simulink model "Navion_6DoF_YANG"  (Simulink 10.3)
settings: Solver=ode45  StartTime=0.0  StopTime=100.0  FixedStep=.01  MaxStep=.004  RelTol=1e-5  EnableMultiTasking=on
values from neighbouring files (symbols this model uses):
  ac = [0 0 0]    [Navion_Geom6dof.m]
  b = 44    [Navion_Geom6dof.m]
  cbar = 4+2/12    (= 4.16666666667)    [Navion_Geom6dof.m]
  cda2 = 0.33    [Navion_Geom6dof.m]
  cdo = 0.05    [Navion_Geom6dof.m]
  cg = [0 0 0]    [Navion_Geom6dof.m]
  cla = 4.44    [Navion_Geom6dof.m]
  cladot = 0    [Navion_Geom6dof.m]
  clb = -0.074    [Navion_Geom6dof.m]
  clda = -0.134    [Navion_Geom6dof.m]
  clde = 0.355    [Navion_Geom6dof.m]
  cldr = 0.107    [Navion_Geom6dof.m]
  clo = 0.41    [Navion_Geom6dof.m]
  clp = -0.410    (= -0.41)    [Navion_Geom6dof.m]
  clq = 3.8    [Navion_Geom6dof.m]
  clr = 0.107    [Navion_Geom6dof.m]
  cma = -0.683    [Navion_Geom6dof.m]
  cmadot = -4.36    [Navion_Geom6dof.m]
  cmde = -0.923    [Navion_Geom6dof.m]
  cmq = -9.96    [Navion_Geom6dof.m]
  cnb = 0.071    [Navion_Geom6dof.m]
  cnda = -0.0035    [Navion_Geom6dof.m]
  cndr = -0.072    [Navion_Geom6dof.m]
  cnp = -0.0575    [Navion_Geom6dof.m]
  cnr = -0.125    [Navion_Geom6dof.m]
  cyb = -0.564    [Navion_Geom6dof.m]
  cydr = 0.157    [Navion_Geom6dof.m]
  initalt = 6000    [Navion_Geom6dof.m]
  initbank = 0    [Navion_Geom6dof.m]
  initeast = 0    [Navion_Geom6dof.m]
  inithead = 0    [Navion_Geom6dof.m]
  initnorth = 0    [Navion_Geom6dof.m]
  initp = 0    [Navion_Geom6dof.m]
  initpitch = initw/initu    (= -0.0290599038041)    [Navion_Geom6dof.m]
  initq = 0    [Navion_Geom6dof.m]
  initr = 0    [Navion_Geom6dof.m]
  initu = 228.7    [Navion_Geom6dof.m]
  initv = 0    [Navion_Geom6dof.m]
  initw = -6.646    [Navion_Geom6dof.m]
  jx = 1048    [Navion_Geom6dof.m]
  jxz = 0    [Navion_Geom6dof.m]
  jy = 3000    [Navion_Geom6dof.m]
  jz = 3500    [Navion_Geom6dof.m]
  Pos_L = [95.46/12-3.882,5.1875,0]    [Navion_Geom6dof.m]
  Pos_R = [95.46/12,-5.1875,0]    [Navion_Geom6dof.m]
  sw = 175.3    [Navion_Geom6dof.m]
  Vect_L = [0.998,-0.057,0.017]    [Navion_Geom6dof.m]
  Vect_R = [0.998,0.057,0.017]    [Navion_Geom6dof.m]
  weight = 3695    [Navion_Geom6dof.m]
undefined symbols (not defined in the file or in its folder): BHP_A, BHP_B, CP_norm, Pr_Alt, PropEff_norm
libraries: simulink_extras x4, aerolibatmos2 x2
(part 1 of 2)
settings Model: Creator=andersop  LastModifiedBy=YANGX5  MultithreadedSim=on  ExtModeAutoUpdateStatusClock=off
settings SolverCC: InitialStep=.004
settings DataIOCC: LimitDataPoints=on  SaveState=on  SignalLoggingName=sigsOut
settings OptimizationCC: InitFltsAndDblsToZero=on
settings DebuggingCC: SaveWithParameterizedLinksMsg=none  SignalResolutionControl=TryResolveAllWithWarning  MultiTaskDSMMsg=warning  MultiTaskCondExecSysMsg=none
settings HardwareCC: TargetUnknown=on
settings GRTTargetCC: TargetFcnLib=ansi_tfl_tmw.mat  ModelReferenceCompliant=off  MatFileLogging=off

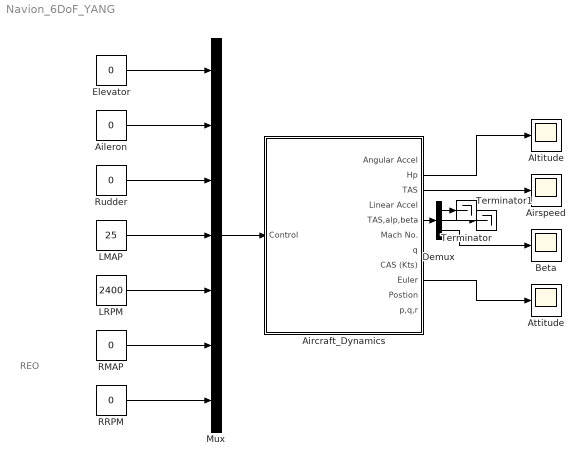
== system Navion_6DoF_YANG ==
  note: REO
  Aileron : Constant  Value=0
  Aircraft_Dynamics : Subsystem
  Airspeed : Scope
  Altitude : Scope
  Attitude : Scope
  Beta : Scope
  Demux : Demux  Outputs=3
  Elevator : Constant  Value=0
  LMAP : Constant  Value=25
  LRPM : Constant  Value=2400
  Mux : Mux  Inputs=7
  RMAP : Constant  Value=0
  RRPM : Constant  Value=0
  Rudder : Constant  Value=0
  Terminator : Terminator
  Terminator1 : Terminator
  wires:
  Mux/1 -> Aircraft_Dynamics/1(Control)
  Elevator/1 -> Mux/1
  LRPM/1 -> Mux/5
  RMAP/1 -> Mux/6
  RRPM/1 -> Mux/7
  Aileron/1 -> Mux/2
  Rudder/1 -> Mux/3
  LMAP/1 -> Mux/4
  Aircraft_Dynamics/2(Hp) -> Altitude/1
  Aircraft_Dynamics/3(TAS) -> Airspeed/1
  Aircraft_Dynamics/9(Euler) -> Attitude/1
  Aircraft_Dynamics/5(TAS,alp,beta) -> Demux/1
  Demux/3 -> Beta/1
  Demux/1 -> Terminator/1
  Demux/2 -> Terminator1/1

== system Navion_6DoF_YANG/Aircraft_Dynamics ==
  Control : Inport
  Aerodynamics : Subsystem
  Display : Display
  Engines : Subsystem
  "Equations of motion numerical integration " : Subsystem
  Flight Parameters : Subsystem
  Linear Acc and Moments : Subsystem
  "Mass, CG & inertia" : Subsystem
  Standard Atmosphere : Subsystem
  Angular Accel : Outport
  Hp : Outport  Port=2
  TAS : Outport  Port=3
  Linear Accel : Outport  Port=4
  TAS,alp,beta : Outport  Port=5
  Mach No. : Outport  Port=6
  q : Outport  Port=7
  CAS (Kts) : Outport  Port=8
  Euler : Outport  Port=9
  Postion : Outport  Port=10
  p,q,r : Outport  Port=11
  wires:
  Aerodynamics/1(Faero) -> Linear Acc and Moments/1(Faero)
  Aerodynamics/2(Maero) -> Linear Acc and Moments/2(Maero)
  Control/1 -> Aerodynamics/3(Controls), Engines/1(Control)
  "Mass, CG & inertia"/1(CG) -> Linear Acc and Moments/6(CG)
  "Mass, CG & inertia"/2(Inertia) -> "Equations of motion numerical integration "/2(Inertia)
  Linear Acc and Moments/1(Lin Accel) -> Linear Accel/1, "Equations of motion numerical integration "/1(Accel)
  Linear Acc and Moments/2(Moments) -> "Equations of motion numerical integration "/3(Moments)
  "Equations of motion numerical integration "/3(Ang rates) -> Aerodynamics/6(p,q,r), p,q,r/1
  "Equations of motion numerical integration "/4(Wind Vel) -> Flight Parameters/1(Wind Vel), Display/1
  Flight Parameters/1(Wing Para) -> TAS,alp,beta/1, Aerodynamics/1(Wind Para), Engines/2(Wind Par)
  Flight Parameters/4(Dyn (q)) -> Aerodynamics/2(dyn(q)), q/1
  Flight Parameters/3(Mach No.) -> Mach No./1, Aerodynamics/4(Mach No.)
  Flight Parameters/2(A&Bdot) -> Aerodynamics/5(a&bdot)
  "Equations of motion numerical integration "/2(Position) -> Postion/1, Standard Atmosphere/1(Position)
  "Equations of motion numerical integration "/1(Ang Accel) -> Angular Accel/1
  Standard Atmosphere/4(Hp) -> Engines/3(Hp), Hp/1
  Flight Parameters/5(TAS fps) -> TAS/1
  Flight Parameters/6(CAS(kts)) -> CAS (Kts)/1
  "Equations of motion numerical integration "/5(Euler) -> Euler/1
  Standard Atmosphere/3(a) -> Flight Parameters/2(a)
  Standard Atmosphere/2(rho) -> Flight Parameters/3(rho)
  "Mass, CG & inertia"/3(mass) -> Linear Acc and Moments/5(Mass)
  Standard Atmosphere/1(OAT) -> Engines/4(OTA)
  Engines/1(Feng_L) -> Linear Acc and Moments/3(Feng_L)
  Engines/2(Feng_R) -> Linear Acc and Moments/4(Feng_R)

== system Navion_6DoF_YANG/Aircraft_Dynamics/Aerodynamics ==
  note: Notes: alpha is measured from
  Wind Para : Inport
  dyn(q) : Inport  Port=2
  Controls : Inport  Port=3
  Mach No. : Inport  Port=4
  a&bdot : Inport  Port=5
  p,q,r : Inport  Port=6
  Aero Forces and Moments : Subsystem
  CD : Subsystem
  CL : Subsystem
  CM : Subsystem
  CN : Subsystem
  CY : Subsystem
  Croll : Subsystem
  Faero : Outport
  Maero : Outport  Port=2
  wires:
  Wind Para/1 -> CL/1(Wind Parameters), CY/1(Wind Parameters), Aero Forces and Moments/5(Wind Para), CN/1(Wind Parameters), Croll/1(Wind Parameters), CM/1(Wind Parameters), CD/1(Wind Parameters)
  CL/1(CL) -> Aero Forces and Moments/4(CL)
  Mach No./1 -> CM/3(Mach No.), CN/3(Mach No.), Croll/3(Mach No.), CY/3(Mach No.), CL/3(Mach No.), CD/3(Mach No.)
  a&bdot/1 -> CL/4(a&bdot), CM/4(a&bdot)
  p,q,r/1 -> CM/5(P,q,r), CN/4(P,q,r), Croll/4(P,q,r), CY/4(P,q,r), CL/5(P,q,r)
  Controls/1 -> CM/2(Controls), CD/2(Controls), CN/2(Controls), Croll/2(Controls), CY/2(Controls), CL/2(Controls)
  CD/1(CD) -> Aero Forces and Moments/2(CD)
  CN/1(CN) -> Aero Forces and Moments/8(CN)
  Croll/1(Croll) -> Aero Forces and Moments/6(Croll)
  CY/1(CY) -> Aero Forces and Moments/3(CY)
  CM/1(CM) -> Aero Forces and Moments/7(CM)
  dyn(q)/1 -> Aero Forces and Moments/1(dyn(q))
  Aero Forces and Moments/1(Faero) -> Faero/1
  Aero Forces and Moments/2(Maero) -> Maero/1

== system Navion_6DoF_YANG/Aircraft_Dynamics/Engines ==
  Control : Inport
  Wind Par : Inport  Port=2
  Hp : Inport  Port=3
  OTA : Inport  Port=4
  Demux : Demux  Outputs=7
  Demux1 : Demux  Outputs=3
  Display : Display
  Display1 : Display
  Lycoming IO-Left : Subsystem
  Lycoming IO-Right : Subsystem
  Terminator{,1..4} (5 alike) : Terminator
  Feng_L : Outport
  Feng_R : Outport  Port=2
  tag scope: TAS=global
  wires:
  Control/1 -> Demux/1
  Demux/1 -> Terminator/1
  Demux/2 -> Terminator1/1
  Demux/3 -> Terminator2/1
  Lycoming IO-Left/1(Thrust Left) -> Feng_L/1, Display/1
  Wind Par/1 -> Demux1/1
  Demux1/2 -> Terminator4/1
  Demux1/3 -> Terminator3/1
  Lycoming IO-Right/1(Thrust right) -> Feng_R/1, Display1/1
  Demux/4 -> Lycoming IO-Left/1(MAP_L)
  Demux/5 -> Lycoming IO-Left/2(RPM_L)
  Demux/6 -> Lycoming IO-Right/1(MAP_R)
  Demux/7 -> Lycoming IO-Right/2(RPM_R)
  Hp/1 -> Lycoming IO-Right/3(Press alt), Lycoming IO-Left/3(Press alt)
  OTA/1 -> Lycoming IO-Right/4(Inlt Temp), Lycoming IO-Left/4(Inlt Temp)
  Demux1/1 -> [TAS]  "TAS"

== system Navion_6DoF_YANG/Aircraft_Dynamics/Equations of motion numerical integration  ==
  Accel : Inport
  Inertia : Inport  Port=2
  Moments : Inport  Port=3
  Flat Earth Navigation : Subsystem
  Force Equations : Subsystem
  Gravity Model : Subsystem
  Inert-body : Subsystem
  Kinematic Equiations : Subsystem
  Moment Equations : Subsystem
  Ang Accel : Outport
  Position : Outport  Port=2
  Ang rates : Outport  Port=3
  Wind Vel : Outport  Port=4
  Euler : Outport  Port=5
  wires:
  Moment Equations/1(Ang Rates) -> Kinematic Equiations/1(Rates), Force Equations/3(Rates), Ang rates/1
  Kinematic Equiations/1(Euler angles) -> Flat Earth Navigation/1(Euler Angles), Inert-body/1(Euler), Euler/1
  Force Equations/1(Lin Vel) -> Wind Vel/1, Flat Earth Navigation/2(Velocity)
  Accel/1 -> Force Equations/1(Accel)
  Inertia/1 -> Moment Equations/1(Inertia)
  Gravity Model/1(Gravity) -> Force Equations/2(Gravity)
  Moments/1 -> Moment Equations/2(Moments)
  Moment Equations/2(Ang Accel) -> Ang Accel/1
  Flat Earth Navigation/1(Position) -> Position/1
  Inert-body/1(NEDtoBC) -> Force Equations/4(NEDtoABC)

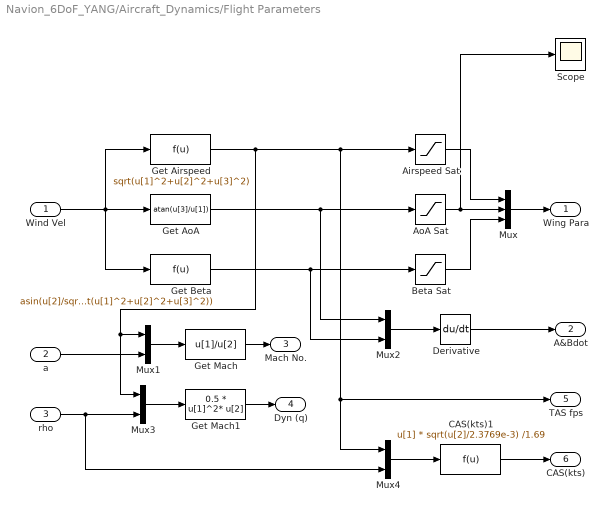
== system Navion_6DoF_YANG/Aircraft_Dynamics/Flight Parameters ==
  Wind Vel : Inport
  a : Inport  Port=2
  rho : Inport  Port=3
  Airspeed Sat : Saturate  UpperLimit=1100  LowerLimit=0
  AoA Sat : Saturate  UpperLimit=0.3  LowerLimit=-0.2
  Beta Sat : Saturate  UpperLimit=0.4  LowerLimit=-0.4
  CAS(kts)1 : Fcn  Expr=u[1] * sqrt(u[2]/2.3769e-3) /1.69
  Derivative : Derivative
  Get Airspeed : Fcn  Expr=sqrt(u[1]^2+u[2]^2+u[3]^2)
  Get AoA : Fcn  Expr=atan(u[3]/u[1])
  Get Beta : Fcn  Expr=asin(u[2]/sqrt(u[1]^2+u[2]^2+u[3]^2))
  Get Mach : Fcn  Expr=u[1]/u[2]
  Get Mach1 : Fcn  Expr=0.5 * u[1]^2* u[2]
  Mux : Mux  Inputs=3
  Mux{1..4} (4 alike) : Mux  Inputs=2
  Scope : Scope
  Wing Para : Outport
  A&Bdot : Outport  Port=2
  Mach No. : Outport  Port=3
  Dyn (q) : Outport  Port=4
  TAS fps : Outport  Port=5
  CAS(kts) : Outport  Port=6
  wires:
  Wind Vel/1 -> Get AoA/1, Get Airspeed/1, Get Beta/1
  Get Airspeed/1 -> Mux1/1, Mux3/1, Airspeed Sat/1, TAS fps/1, Mux4/1
  Get AoA/1 -> AoA Sat/1, Mux2/1
  Get Beta/1 -> Beta Sat/1, Mux2/2
  AoA Sat/1 -> Mux/2, Scope/1
  Airspeed Sat/1 -> Mux/1
  Beta Sat/1 -> Mux/3
  Mux/1 -> Wing Para/1
  Mux1/1 -> Get Mach/1
  a/1 -> Mux1/2
  Mux2/1 -> Derivative/1
  Derivative/1 -> A&Bdot/1
  Get Mach/1 -> Mach No./1
  rho/1 -> Mux3/2, Mux4/2
  Mux3/1 -> Get Mach1/1
  Get Mach1/1 -> Dyn (q)/1
  Mux4/1 -> CAS(kts)1/1
  CAS(kts)1/1 -> CAS(kts)/1

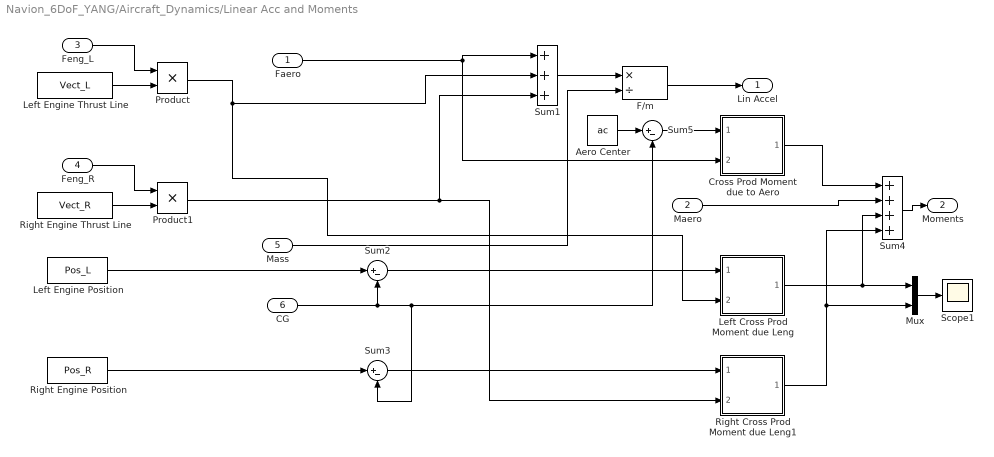
== system Navion_6DoF_YANG/Aircraft_Dynamics/Linear Acc and Moments ==
  Faero : Inport
  Maero : Inport  Port=2
  Feng_L : Inport  Port=3
  Feng_R : Inport  Port=4
  Mass : Inport  Port=5
  CG : Inport  Port=6
  Aero Center : Constant  Value=ac
  Cross Prod Moment due to Aero : Subsystem
  F/m : Product  Inputs=*/  SaturateOnIntegerOverflow=on  OutDataTypeStr=Inherit: Same as first input
  Left Cross Prod Moment due Leng : Subsystem
  Left Engine Position : Constant  Value=Pos_L
  Left Engine Thrust Line : Constant  Value=Vect_L
  Mux : Mux  Inputs=2
  Product : Product
  Product1 : Product
  Right Cross Prod Moment due Leng1 : Subsystem
  Right Engine Position : Constant  Value=Pos_R
  Right Engine Thrust Line : Constant  Value=Vect_R
  Scope1 : Scope
  Sum1 : Sum  Inputs=+++  SaturateOnIntegerOverflow=on
  Sum2 : Sum  Inputs=|+-  SaturateOnIntegerOverflow=on
  Sum3 : Sum  Inputs=|+-  SaturateOnIntegerOverflow=on
  Sum4 : Sum  Inputs=++++  SaturateOnIntegerOverflow=on
  Sum5 : Sum  Inputs=|+-  SaturateOnIntegerOverflow=on
  Lin Accel : Outport
  Moments : Outport  Port=2
  wires:
  Product/1 -> Sum1/2, Left Cross Prod Moment due Leng/2(Vec 2)
  Faero/1 -> Sum1/1, Cross Prod Moment due to Aero/2(Vec 2)
  Sum1/1 -> F/m/1
  Mass/1 -> F/m/2
  F/m/1 -> Lin Accel/1
  Aero Center/1 -> Sum5/1
  Sum5/1 -> Cross Prod Moment due to Aero/1(Vec 1)
  Maero/1 -> Sum4/2
  Sum4/1 -> Moments/1
  Cross Prod Moment due to Aero/1(X Prod) -> Sum4/1
  Sum2/1 -> Left Cross Prod Moment due Leng/1(Vec 1)
  Left Cross Prod Moment due Leng/1(X Prod) -> Mux/1, Sum4/3
  Left Engine Position/1 -> Sum2/1
  Feng_L/1 -> Product/1
  Left Engine Thrust Line/1 -> Product/2
  Feng_R/1 -> Product1/1
  Right Engine Thrust Line/1 -> Product1/2
  Right Engine Position/1 -> Sum3/1
  CG/1 -> Sum2/2, Sum3/2, Sum5/2
  Sum3/1 -> Right Cross Prod Moment due Leng1/1(Vec 1)
  Product1/1 -> Sum1/3, Right Cross Prod Moment due Leng1/2(Vec 2)
  Right Cross Prod Moment due Leng1/1(X Prod) -> Mux/2, Sum4/4
  Mux/1 -> Scope1/1

== system Navion_6DoF_YANG/Aircraft_Dynamics/Mass, CG & inertia ==
  Mux1 : Mux
  cg : Constant  Value=cg
  jx : Constant  Value=jx
  jxz : Constant  Value=jxz
  jy : Constant  Value=jy
  jz : Constant  Value=jz
  mass2 : Constant  Value=weight/32.2
  CG : Outport
  Inertia : Outport  Port=2
  mass : Outport  Port=3
  wires:
  cg/1 -> CG/1
  jy/1 -> Mux1/2
  jx/1 -> Mux1/1
  jz/1 -> Mux1/3
  jxz/1 -> Mux1/4
  Mux1/1 -> Inertia/1
  mass2/1 -> mass/1

== system Navion_6DoF_YANG/Aircraft_Dynamics/Standard Atmosphere ==
  Position : Inport
  Demux : Demux  Outputs=3
      settings: DisplayOption=none
  Density : Fcn  Expr=2.3769e-3*(1 - 0.703e-5 * u[1])^4.14
  OATemp : Lookup  InputValues=[0 35000 60000]  Table=[519 390 390]  SaturateOnIntegerOverflow=on
  Speed of Sound : Fcn  Expr=sqrt(1.4*1716.3*u[1])
  Terminator : Terminator
  Terminator1 : Terminator
  OAT : Outport
  rho : Outport  Port=2
  a : Outport  Port=3
  Hp : Outport  Port=4
  wires:
  OATemp/1 -> OAT/1, Speed of Sound/1
  Density/1 -> rho/1
  Speed of Sound/1 -> a/1
  Position/1 -> Demux/1
  Demux/1 -> Terminator/1
  Demux/2 -> Terminator1/1
  Demux/3 -> OATemp/1, Density/1, Hp/1

== system Navion_6DoF_YANG/Aircraft_Dynamics/Aerodynamics/Aero Forces and Moments ==
  dyn(q) : Inport
  CD : Inport  Port=2
  CY : Inport  Port=3
  CL : Inport  Port=4
  Wind Para : Inport  Port=5
  Croll : Inport  Port=6
  CM : Inport  Port=7
  CN : Inport  Port=8
  Aerodynamic Forces : Subsystem
  Aerodynamic Moments : Subsystem
  Faero : Outport
  Maero : Outport  Port=2
  wires:
  dyn(q)/1 -> Aerodynamic Moments/1(dyn(q)), Aerodynamic Forces/5(dyn(q))
  CD/1 -> Aerodynamic Forces/1(CD)
  CY/1 -> Aerodynamic Forces/2(CY)
  CL/1 -> Aerodynamic Forces/3(CL)
  Wind Para/1 -> Aerodynamic Forces/4(Wind Para)
  Croll/1 -> Aerodynamic Moments/2(Croll)
  CM/1 -> Aerodynamic Moments/3(CM)
  CN/1 -> Aerodynamic Moments/4(CN)
  Aerodynamic Forces/1(FaeroBody) -> Faero/1
  Aerodynamic Moments/1(Maero) -> Maero/1

== system Navion_6DoF_YANG/Aircraft_Dynamics/Aerodynamics/CD ==
  Wind Parameters : Inport
  Controls : Inport  Port=2
  Mach No. : Inport  Port=3
  "   1" : Terminator
  "   6" : Terminator
  Get Alpha : Subsystem
  Math Function : Math  Operator=square  SignedPower=on  SaturateOnIntegerOverflow=on
  Sum : Sum  SaturateOnIntegerOverflow=on
  cda2 : Gain  Gain=cda2  SaturateOnIntegerOverflow=on  OutDataTypeStr=Inherit: Same as input  ParamDataTypeStr=Inherit: Same as input
  cdo : Constant  Value=cdo
  CD : Outport
  wires:
  Wind Parameters/1 -> Get Alpha/1(windPar)
  Sum/1 -> CD/1
  Controls/1 -> "   6"/1
  Get Alpha/1(Alpha) -> Math Function/1
  Math Function/1 -> cda2/1
  cda2/1 -> Sum/2
  Mach No./1 -> "   1"/1
  cdo/1 -> Sum/1

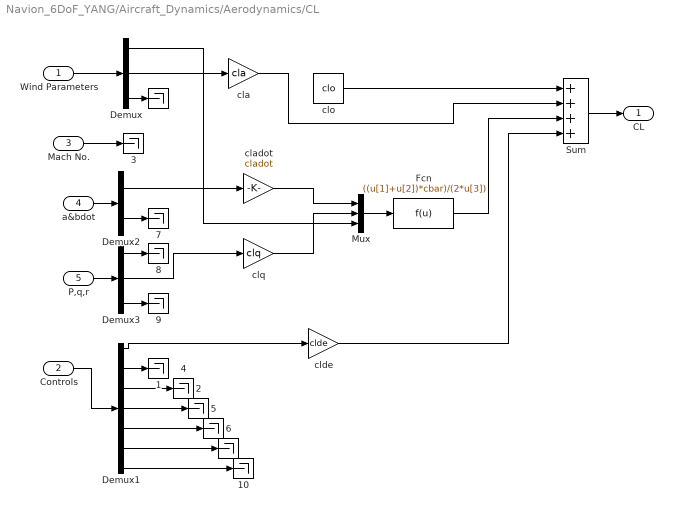
== system Navion_6DoF_YANG/Aircraft_Dynamics/Aerodynamics/CL ==
  Wind Parameters : Inport
  Controls : Inport  Port=2
  Mach No. : Inport  Port=3
  a&bdot : Inport  Port=4
  P,q,r : Inport  Port=5
     {,1..10} (11 alike) : Terminator
  Demux : Demux  Outputs=3
      settings: DisplayOption=none
  Demux1 : Demux  Outputs=7
      settings: DisplayOption=none
  Demux2 : Demux  Outputs=2
      settings: DisplayOption=none
  Demux3 : Demux  Outputs=3
      settings: DisplayOption=none
  Fcn : Fcn  Expr=((u[1]+u[2])*cbar)/(2*u[3])
  Mux : Mux  Inputs=3
  Sum : Sum  Inputs=++++  SaturateOnIntegerOverflow=on
  cla : Gain  Gain=cla  SaturateOnIntegerOverflow=on  OutDataTypeStr=Inherit: Same as input  ParamDataTypeStr=Inherit: Same as input
  cladot : Gain  Gain=cladot  SaturateOnIntegerOverflow=on  OutDataTypeStr=Inherit: Same as input  ParamDataTypeStr=Inherit: Same as input
  clde : Gain  Gain=clde  SaturateOnIntegerOverflow=on  OutDataTypeStr=Inherit: Same as input  ParamDataTypeStr=Inherit: Same as input
  clo : Constant  Value=clo
  clq : Gain  Gain=clq  SaturateOnIntegerOverflow=on  OutDataTypeStr=Inherit: Same as input  ParamDataTypeStr=Inherit: Same as input
  CL : Outport
  wires:
  Mux/1 -> Fcn/1
  Demux/1 -> Mux/3
  clo/1 -> Sum/1
  Demux2/2 -> "   7"/1
  Demux3/1 -> "   8"/1
  Demux3/3 -> "   9"/1
  Wind Parameters/1 -> Demux/1
  Sum/1 -> CL/1
  Controls/1 -> Demux1/1
  a&bdot/1 -> Demux2/1
  P,q,r/1 -> Demux3/1
  Demux/3 -> "   "/1
  Demux1/4 -> "   2"/1
  cla/1 -> Sum/2
  Demux2/1 -> cladot/1
  cladot/1 -> Mux/1
  Demux/2 -> cla/1
  clq/1 -> Mux/2
  Mach No./1 -> "   3"/1
  Demux3/2 -> clq/1
  Demux1/1 -> clde/1
  Demux1/2 -> "   1"/1
  Demux1/3 -> "   4"/1
  Fcn/1 -> Sum/3
  clde/1 -> Sum/4
  Demux1/5 -> "   5"/1
  Demux1/6 -> "   6"/1
  Demux1/7 -> "   10"/1

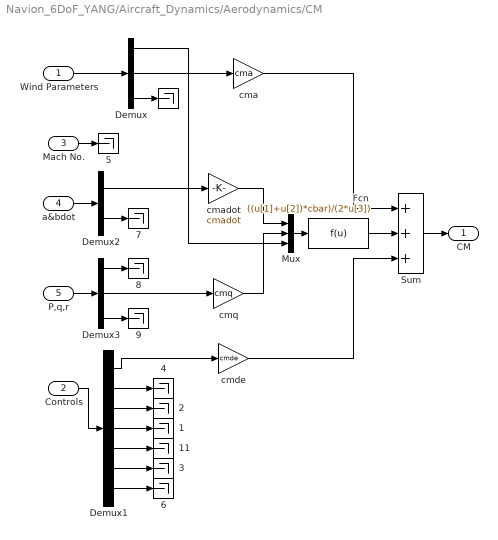
== system Navion_6DoF_YANG/Aircraft_Dynamics/Aerodynamics/CM ==
  Wind Parameters : Inport
  Controls : Inport  Port=2
  Mach No. : Inport  Port=3
  a&bdot : Inport  Port=4
  P,q,r : Inport  Port=5
     {,1..9,11} (11 alike) : Terminator
  Demux : Demux  Outputs=3
      settings: DisplayOption=none
  Demux1 : Demux  Outputs=7
      settings: DisplayOption=none
  Demux2 : Demux  Outputs=2
      settings: DisplayOption=none
  Demux3 : Demux  Outputs=3
      settings: DisplayOption=none
  Fcn : Fcn  Expr=((u[1]+u[2])*cbar)/(2*u[3])
  Mux : Mux  Inputs=3
  Sum : Sum  Inputs=+++  SaturateOnIntegerOverflow=on
  cma : Gain  Gain=cma  SaturateOnIntegerOverflow=on  OutDataTypeStr=Inherit: Same as input  ParamDataTypeStr=Inherit: Same as input
  cmadot : Gain  Gain=cmadot  SaturateOnIntegerOverflow=on  OutDataTypeStr=Inherit: Same as input  ParamDataTypeStr=Inherit: Same as input
  cmde : Gain  Gain=cmde  SaturateOnIntegerOverflow=on  OutDataTypeStr=Inherit: Same as input  ParamDataTypeStr=Inherit: Same as input
  cmq : Gain  Gain=cmq  SaturateOnIntegerOverflow=on  OutDataTypeStr=Inherit: Same as input  ParamDataTypeStr=Inherit: Same as input
  CM : Outport
  wires:
  Demux2/2 -> "   7"/1
  Demux3/1 -> "   8"/1
  Demux3/3 -> "   9"/1
  Wind Parameters/1 -> Demux/1
  Sum/1 -> CM/1
  Controls/1 -> Demux1/1
  a&bdot/1 -> Demux2/1
  P,q,r/1 -> Demux3/1
  Demux/3 -> "   "/1
  Demux1/4 -> "   1"/1
  Demux1/3 -> "   2"/1
  Demux/2 -> cma/1
  cmadot/1 -> Mux/1
  cmq/1 -> Mux/2
  Mux/1 -> Fcn/1
  Demux1/2 -> "   4"/1
  Mach No./1 -> "   5"/1
  Demux/1 -> Mux/3
  cma/1 -> Sum/1
  Demux1/1 -> cmde/1
  Demux2/1 -> cmadot/1
  Demux3/2 -> cmq/1
  Fcn/1 -> Sum/2
  cmde/1 -> Sum/3
  Demux1/5 -> "   11"/1
  Demux1/6 -> "   3"/1
  Demux1/7 -> "   6"/1

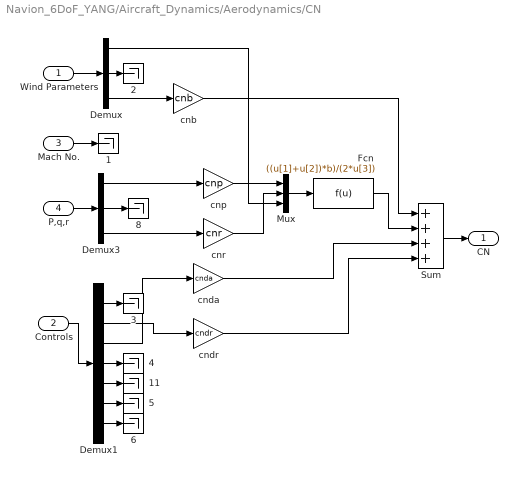
== system Navion_6DoF_YANG/Aircraft_Dynamics/Aerodynamics/CN ==
  Wind Parameters : Inport
  Controls : Inport  Port=2
  Mach No. : Inport  Port=3
  P,q,r : Inport  Port=4
     {1..6,8,11} (8 alike) : Terminator
  Demux : Demux  Outputs=3
      settings: DisplayOption=none
  Demux1 : Demux  Outputs=7
      settings: DisplayOption=none
  Demux3 : Demux  Outputs=3
      settings: DisplayOption=none
  Fcn : Fcn  Expr=((u[1]+u[2])*b)/(2*u[3])
  Mux : Mux  Inputs=3
  Sum : Sum  Inputs=++++  SaturateOnIntegerOverflow=on
  cnb : Gain  Gain=cnb  SaturateOnIntegerOverflow=on  OutDataTypeStr=Inherit: Same as input  ParamDataTypeStr=Inherit: Same as input
  cnda : Gain  Gain=cnda  SaturateOnIntegerOverflow=on  OutDataTypeStr=Inherit: Same as input  ParamDataTypeStr=Inherit: Same as input
  cndr : Gain  Gain=cndr  SaturateOnIntegerOverflow=on  OutDataTypeStr=Inherit: Same as input  ParamDataTypeStr=Inherit: Same as input
  cnp : Gain  Gain=cnp  SaturateOnIntegerOverflow=on  OutDataTypeStr=Inherit: Same as input  ParamDataTypeStr=Inherit: Same as input
  cnr : Gain  Gain=cnr  SaturateOnIntegerOverflow=on  OutDataTypeStr=Inherit: Same as input  ParamDataTypeStr=Inherit: Same as input
  CN : Outport
  wires:
  Mux/1 -> Fcn/1
  Demux/2 -> "   2"/1
  Wind Parameters/1 -> Demux/1
  Sum/1 -> CN/1
  Controls/1 -> Demux1/1
  P,q,r/1 -> Demux3/1
  Demux3/2 -> "   8"/1
  cnb/1 -> Sum/1
  Mach No./1 -> "   1"/1
  Demux/3 -> cnb/1
  Demux/1 -> Mux/3
  Demux3/1 -> cnp/1
  cnp/1 -> Mux/1
  Demux3/3 -> cnr/1
  cnr/1 -> Mux/2
  Demux1/2 -> cndr/1
  Demux1/3 -> cnda/1
  Fcn/1 -> Sum/2
  cnda/1 -> Sum/3
  cndr/1 -> Sum/4
  Demux1/1 -> "   3"/1
  Demux1/4 -> "   4"/1
  Demux1/5 -> "   11"/1
  Demux1/6 -> "   5"/1
  Demux1/7 -> "   6"/1

== system Navion_6DoF_YANG/Aircraft_Dynamics/Aerodynamics/CY ==
  Wind Parameters : Inport
  Controls : Inport  Port=2
  Mach No. : Inport  Port=3
  P,q,r : Inport  Port=4
     {1..5,8..12} (10 alike) : Terminator
  Demux : Demux  Outputs=3
      settings: DisplayOption=none
  Demux1 : Demux  Outputs=7
      settings: DisplayOption=none
  Sum : Sum  SaturateOnIntegerOverflow=on
  cyb : Gain  Gain=cyb  SaturateOnIntegerOverflow=on  OutDataTypeStr=Inherit: Same as input  ParamDataTypeStr=Inherit: Same as input
  cydr : Gain  Gain=cydr  SaturateOnIntegerOverflow=on  OutDataTypeStr=Inherit: Same as input  ParamDataTypeStr=Inherit: Same as input
  CY : Outport
  wires:
  Demux/2 -> "   9"/1
  Wind Parameters/1 -> Demux/1
  Sum/1 -> CY/1
  Controls/1 -> Demux1/1
  P,q,r/1 -> "   8"/1
  Demux/3 -> cyb/1
  Mach No./1 -> "   2"/1
  Demux1/1 -> "   10"/1
  Demux1/2 -> cydr/1
  Demux1/4 -> "   11"/1
  cyb/1 -> Sum/1
  cydr/1 -> Sum/2
  Demux/1 -> "   12"/1
  Demux1/3 -> "   1"/1
  Demux1/5 -> "   3"/1
  Demux1/6 -> "   4"/1
  Demux1/7 -> "   5"/1

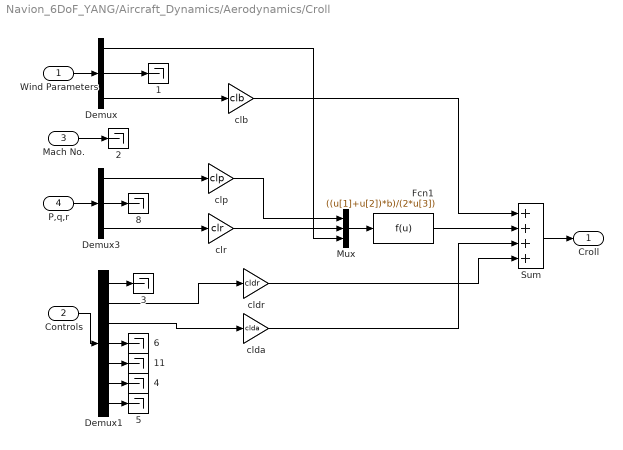
== system Navion_6DoF_YANG/Aircraft_Dynamics/Aerodynamics/Croll ==
  Wind Parameters : Inport
  Controls : Inport  Port=2
  Mach No. : Inport  Port=3
  P,q,r : Inport  Port=4
     {1..6,8,11} (8 alike) : Terminator
  Demux : Demux  Outputs=3
      settings: DisplayOption=none
  Demux1 : Demux  Outputs=7
      settings: DisplayOption=none
  Demux3 : Demux  Outputs=3
      settings: DisplayOption=none
  Fcn1 : Fcn  Expr=((u[1]+u[2])*b)/(2*u[3])
  Mux : Mux  Inputs=3
  Sum : Sum  Inputs=++++  SaturateOnIntegerOverflow=on
  clb : Gain  Gain=clb  SaturateOnIntegerOverflow=on  OutDataTypeStr=Inherit: Same as input  ParamDataTypeStr=Inherit: Same as input
  clda : Gain  Gain=clda  SaturateOnIntegerOverflow=on  OutDataTypeStr=Inherit: Same as input  ParamDataTypeStr=Inherit: Same as input
  cldr : Gain  Gain=cldr  SaturateOnIntegerOverflow=on  OutDataTypeStr=Inherit: Same as input  ParamDataTypeStr=Inherit: Same as input
  clp : Gain  Gain=clp  SaturateOnIntegerOverflow=on  OutDataTypeStr=Inherit: Same as input  ParamDataTypeStr=Inherit: Same as input
  clr : Gain  Gain=clr  SaturateOnIntegerOverflow=on  OutDataTypeStr=Inherit: Same as input  ParamDataTypeStr=Inherit: Same as input
  Croll : Outport
  wires:
  Mux/1 -> Fcn1/1
  Demux/2 -> "   1"/1
  Wind Parameters/1 -> Demux/1
  Sum/1 -> Croll/1
  Controls/1 -> Demux1/1
  P,q,r/1 -> Demux3/1
  Demux3/2 -> "   8"/1
  Demux1/1 -> "   3"/1
  clp/1 -> Mux/1
  clb/1 -> Sum/1
  Demux/1 -> Mux/3
  Demux/3 -> clb/1
  Mach No./1 -> "   2"/1
  Demux3/1 -> clp/1
  Fcn1/1 -> Sum/2
  Demux3/3 -> clr/1
  clr/1 -> Mux/2
  Demux1/4 -> "   6"/1
  Demux1/2 -> cldr/1
  Demux1/3 -> clda/1
  clda/1 -> Sum/3
  cldr/1 -> Sum/4
  Demux1/5 -> "   11"/1
  Demux1/6 -> "   4"/1
  Demux1/7 -> "   5"/1

== system Navion_6DoF_YANG/Aircraft_Dynamics/Engines/Lycoming IO-Left ==
  MAP_L : Inport
  RPM_L : Inport  Port=2
  Press alt : Inport  Port=3
  Inlt Temp : Inport  Port=4
  Prop Efficiency  with Cp input : Subsystem
  Subsystem : Subsystem
  Thrust : Subsystem
  Thrust Left : Outport
  tag scope: Cp_left=global
  wires:
  Inlt Temp/1 -> Subsystem/4(Inlet temp C)
  Press alt/1 -> Subsystem/3(Pressure alt)
  Thrust/1("thrust ") -> Thrust Left/1
  RPM_L/1 -> Subsystem/2(RPM1)
  MAP_L/1 -> Subsystem/1(Map)
  Subsystem/1(Cp) -> [Cp_left]
  Prop Efficiency  with Cp input/1(n) -> [n]
  [n] -> Thrust/3(n)
  [BHP_E_left] -> Thrust/2(BHP E)
  [Prop_D_left] -> Prop Efficiency  with Cp input/3(Prop D)
  [RPS_left] -> Prop Efficiency  with Cp input/2(RPS)
  [TAS] -> Prop Efficiency  with Cp input/1(TAS)
  [TAS] -> Thrust/1(TAS)

== system Navion_6DoF_YANG/Aircraft_Dynamics/Engines/Lycoming IO-Right ==
  MAP_R : Inport
  RPM_R : Inport  Port=2
  Press alt : Inport  Port=3
  Inlt Temp : Inport  Port=4
  Prop Efficiency  with Cp input : Subsystem
  Subsystem : Subsystem
  Thrust : Subsystem
  Thrust right : Outport
  tag scope: Cp_right=global
  wires:
  Inlt Temp/1 -> Subsystem/4(Inlet temp C)
  Press alt/1 -> Subsystem/3(Pressure alt)
  Thrust/1("thrust ") -> Thrust right/1
  RPM_R/1 -> Subsystem/2(RPM1)
  MAP_R/1 -> Subsystem/1(Map)
  Subsystem/1(Cp) -> [Cp_right]
  Prop Efficiency  with Cp input/1(n) -> [n]
  [n] -> Thrust/3(n)
  [BHP_E_right] -> Thrust/2(BHP E)
  [Prop_D_right] -> Prop Efficiency  with Cp input/3(Prop D)
  [RPS_right] -> Prop Efficiency  with Cp input/2(RPS)
  [TAS] -> Prop Efficiency  with Cp input/1(TAS)
  [TAS] -> Thrust/1(TAS)

== system Navion_6DoF_YANG/Aircraft_Dynamics/Equations of motion numerical integration /Flat Earth Navigation ==
  note: 1  roll
      | 2  pitch
      | 3  yaw
      | 4 u
      | 5 v
      | 6 w
  Euler Angles : Inport
  Velocity : Inport  Port=2
  Alt : Integrator  InitialCondition=initalt
  Alttitude Dot : Fcn  Expr=u[4] * sin(u[2]) - u[5] * sin(u[1]) * cos(u[2]) - u[6] * cos(u[1]) * cos(u[2])
  Demux : Demux  Outputs=3
      settings: DisplayOption=none
  Demux1 : Demux  Outputs=3
      settings: DisplayOption=none
  East : Integrator  InitialCondition=initeast
  East Dot : Fcn  Expr=u[4] * cos(u[2])* sin(u[3]) + u[5] * (cos(u[1])*cos(u[3]) + sin(u[1])*sin(u[2])*sin(u[3])) + u[6] * (-sin(u[1])*cos(u[3])+cos(u[1])*sin(u[2])*sin(u[3]))
  Mux : Mux  Inputs=6
  Mux1 : Mux  Inputs=3
  North : Integrator  InitialCondition=initnorth
  North Dot : Fcn  Expr=u[4] * cos(u[2]) * cos(u[3]) + u[5]*(-cos(u[1])*sin(u[3])+sin(u[1])*sin(u[2])*sin(u[3]))+u[6]*(sin(u[1])*sin(u[3])+cos(u[1])*sin(u[2])*cos(u[3]))
  Position : Outport
  wires:
  Euler Angles/1 -> Demux/1
  Velocity/1 -> Demux1/1
  Demux/1 -> Mux/1
  Demux/2 -> Mux/2
  Demux/3 -> Mux/3
  Demux1/1 -> Mux/4
  Demux1/2 -> Mux/5
  Demux1/3 -> Mux/6
  Mux/1 -> East Dot/1, Alttitude Dot/1, North Dot/1
  East Dot/1 -> East/1
  North Dot/1 -> North/1
  Alttitude Dot/1 -> Alt/1
  East/1 -> Mux1/2
  North/1 -> Mux1/1
  Alt/1 -> Mux1/3
  Mux1/1 -> Position/1

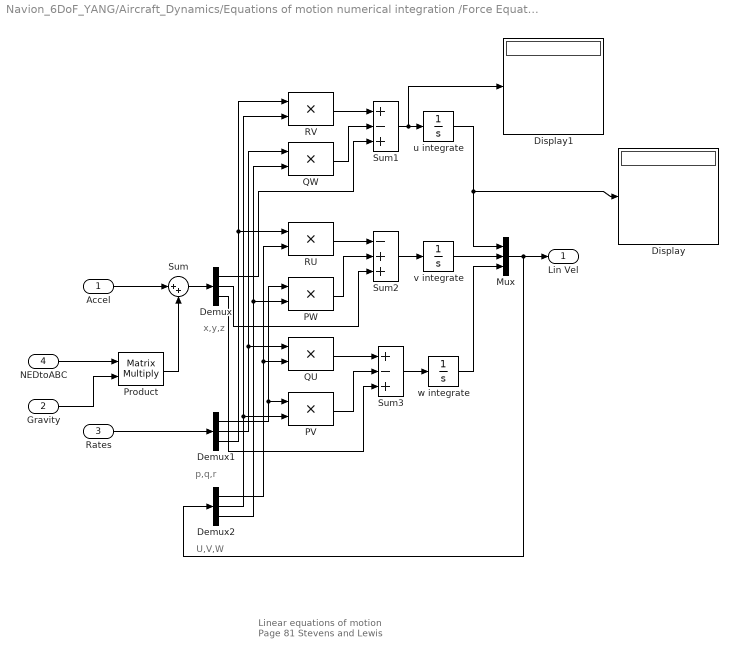
== system Navion_6DoF_YANG/Aircraft_Dynamics/Equations of motion numerical integration /Force Equations ==
  note: U,V,W
  note: p,q,r
  note: x,y,z
  note: Linear equations of motion
      | Page 81 Stevens and Lewis
  Accel : Inport
  Gravity : Inport  Port=2
  Rates : Inport  Port=3
  NEDtoABC : Inport  Port=4
  Demux : Demux  Outputs=3
      settings: DisplayOption=none
  Demux1 : Demux  Outputs=3
      settings: DisplayOption=none
  Demux2 : Demux  Outputs=3
      settings: DisplayOption=none
  Display : Display
  Display1 : Display
  Mux : Mux  Inputs=3
  PV : Product  SaturateOnIntegerOverflow=on  OutDataTypeStr=Inherit: Same as first input
  PW : Product  SaturateOnIntegerOverflow=on  OutDataTypeStr=Inherit: Same as first input
  Product : Product  Multiplication=Matrix(*)  SaturateOnIntegerOverflow=on  OutDataTypeStr=Inherit: Same as first input
  QU : Product  SaturateOnIntegerOverflow=on  OutDataTypeStr=Inherit: Same as first input
  QW : Product  SaturateOnIntegerOverflow=on  OutDataTypeStr=Inherit: Same as first input
  RU : Product  SaturateOnIntegerOverflow=on  OutDataTypeStr=Inherit: Same as first input
  RV : Product  SaturateOnIntegerOverflow=on  OutDataTypeStr=Inherit: Same as first input
  Sum : Sum  Inputs=|++  SaturateOnIntegerOverflow=on
  Sum1 : Sum  Inputs=+-+  SaturateOnIntegerOverflow=on
  Sum2 : Sum  Inputs=-++  SaturateOnIntegerOverflow=on
  Sum3 : Sum  Inputs=+-+  SaturateOnIntegerOverflow=on
  u integrate : Integrator  InitialCondition=initu
  v integrate : Integrator  InitialCondition=initv
  w integrate : Integrator  InitialCondition=initw
  Lin Vel : Outport
  wires:
  Sum/1 -> Demux/1
  Accel/1 -> Sum/1
  Rates/1 -> Demux1/1
  Mux/1 -> Demux2/1, Lin Vel/1
  Demux1/3 -> RV/1, RU/1
  Demux2/2 -> RV/2, PV/2
  RV/1 -> Sum1/1
  Demux1/2 -> QW/1, QU/1
  Demux2/3 -> QW/2, PW/2
  QW/1 -> Sum1/2
  Demux/1 -> Sum1/3
  Demux2/1 -> RU/2, QU/2
  RU/1 -> Sum2/1
  Demux1/1 -> PV/1, PW/1
  PW/1 -> Sum2/2
  Demux/2 -> Sum2/3
  QU/1 -> Sum3/1
  PV/1 -> Sum3/2
  Demux/3 -> Sum3/3
  Gravity/1 -> Product/2
  NEDtoABC/1 -> Product/1
  Product/1 -> Sum/2
  Sum1/1 -> u integrate/1, Display1/1
  Sum2/1 -> v integrate/1
  Sum3/1 -> w integrate/1
  u integrate/1 -> Mux/1, Display/1
  v integrate/1 -> Mux/2
  w integrate/1 -> Mux/3

== system Navion_6DoF_YANG/Aircraft_Dynamics/Equations of motion numerical integration /Gravity Model ==
  Constant : Constant  Value=0
  Constant1 : Constant  Value=32.2
  Mux : Mux  Inputs=3
  Gravity : Outport
  wires:
  Constant/1 -> Mux/1, Mux/2
  Constant1/1 -> Mux/3
  Mux/1 -> Gravity/1

== system Navion_6DoF_YANG/Aircraft_Dynamics/Equations of motion numerical integration /Inert-body ==
  Euler : Inport
  11 : Fcn  Expr=cos(u[2])*cos(u[3])
  12 : Fcn  Expr=-cos(u[1])*sin(u[3])+sin(u[1])*sin(u[2])*cos(u[3])
  13 : Fcn  Expr=sin(u[1])*sin(u[3])+cos(u[1])*sin(u[2])*cos(u[3])
  21 : Fcn  Expr=cos(u[2])*sin(u[3])
  22 : Fcn  Expr=cos(u[1])*cos(u[3]) + sin(u[1])*sin(u[2])*sin(u[3])
  23 : Fcn  Expr=-sin(u[1])*cos(u[3])+cos(u[1])*sin(u[2])*sin(u[3])
  31 : Fcn  Expr=-sin(u[2])
  32 : Fcn  Expr=sin(u[1]) * cos(u[2])
  33 : Fcn  Expr=cos(u[1])*cos(u[2])
  Matrix Concatenation : Concatenate  NumInputs=3  Mode=Multidimensional array
  Matrix Concatenation1 : Concatenate  NumInputs=3  Mode=Multidimensional array
  Matrix Concatenation2 : Concatenate  NumInputs=3  Mode=Multidimensional array
  Matrix Concatenation3 : Concatenate  NumInputs=3  Mode=Multidimensional array  ConcatenateDimension=2
  NEDtoBC : Outport
  wires:
  Euler/1 -> 11/1, 12/1, 13/1, 21/1, 22/1, 23/1, 31/1, 33/1, 32/1
  12/1 -> Matrix Concatenation/2
  11/1 -> Matrix Concatenation/1
  13/1 -> Matrix Concatenation/3
  22/1 -> Matrix Concatenation1/2
  21/1 -> Matrix Concatenation1/1
  23/1 -> Matrix Concatenation1/3
  32/1 -> Matrix Concatenation2/2
  31/1 -> Matrix Concatenation2/1
  33/1 -> Matrix Concatenation2/3
  Matrix Concatenation1/1 -> Matrix Concatenation3/2
  Matrix Concatenation/1 -> Matrix Concatenation3/1
  Matrix Concatenation2/1 -> Matrix Concatenation3/3
  Matrix Concatenation3/1 -> NEDtoBC/1

== system Navion_6DoF_YANG/Aircraft_Dynamics/Equations of motion numerical integration /Kinematic Equiations ==
  note: 1  p
      | 2  q
      | 3  r
      | 4  bank
      | 5 pitch
      | 6 Yaw
  Rates : Inport
  2pi Bound : Subsystem  mask(2pi bound){}
      mask help: Bounds the input angle to [0, 2pi]. When 0 bound is exceeded the output wraps back to 2pi; when the 2pi bound is exceeded the output wraps back to 0.
      mask Help:
      | Bounds the input angle to [0, 2pi]. When 0 bound is exceeded the output wraps back to 2pi; when the 2pi bound is exceeded the output wraps back to 0.
      | <P><B>Input:</B> any angle in radians, from -Inf to Inf;</P>
      | <P><B>Output:</B> an angle in radians between zero and 2pi.</P>
  Demux : Demux  Outputs=3
      settings: DisplayOption=none
  Demux1 : Demux  Outputs=3
      settings: DisplayOption=none
  Demux2 : Demux  Outputs=3
      settings: DisplayOption=none
  Mux : Mux  Inputs=6
  Mux1 : Mux  Inputs=3
  Mux2 : Mux  Inputs=3
  Yaw rate : Fcn  Expr=(u[2] * sin(u[4]) + u[3] * cos(u[4]))/cos(u[5])
  bank : Integrator  InitialCondition=initbank
  heading : Integrator  InitialCondition=inithead
  pi Bound : Subsystem  mask(pi bound){}
      mask help: Bounds the input angle to [-pi, pi]. When -pi bound is exceeded the output wraps back to pi; when the pi bound is exceeded the output wraps back to -pi.
      mask Help:
      | Bounds the input angle to [-pi, pi]. When -pi bound is exceeded the output wraps back to pi; when the pi bound is exceeded the output wraps back to -pi.
      | <P><B>Input:</B> any angle in radians, from -Inf to Inf;</P>
      | <P><B>Output:</B> an angle in radians between -pi and pi.</P>
  pi Bound1 : Subsystem  mask(pi bound){}
      mask help: Bounds the input angle to [-pi, pi]. When -pi bound is exceeded the output wraps back to pi; when the pi bound is exceeded the output wraps back to -pi.
      mask Help:
      | Bounds the input angle to [-pi, pi]. When -pi bound is exceeded the output wraps back to pi; when the pi bound is exceeded the output wraps back to -pi.
      | <P><B>Input:</B> any angle in radians, from -Inf to Inf;</P>
      | <P><B>Output:</B> an angle in radians between -pi and pi.</P>
  pitch : Integrator  InitialCondition=initpitch
  pitch rate : Fcn  Expr=u[2] *cos(u[4]) - u[3] * sin(u[4])
  roll rate : Fcn  Expr=u[1] + tan(u[5])*(u[2]*sin(u[4])+u[3]*cos(u[4]))
  Euler angles : Outport
  wires:
  Rates/1 -> Demux/1
  Demux/2 -> Mux/2
  Demux/3 -> Mux/3
  Demux1/1 -> Mux/4
  Demux1/2 -> Mux/5
  Demux1/3 -> Mux/6
  Demux/1 -> Mux/1
  Mux/1 -> roll rate/1, Yaw rate/1, pitch rate/1
  Demux2/3 -> 2pi Bound/1(In)
  Demux2/2 -> pi Bound/1(In)
  Demux2/1 -> pi Bound1/1(In)
  Mux2/1 -> Euler angles/1
  pi Bound/1(Out) -> Mux2/2
  pi Bound1/1(Out) -> Mux2/1
  2pi Bound/1(Out) -> Mux2/3
  pitch rate/1 -> pitch/1
  roll rate/1 -> bank/1
  Yaw rate/1 -> heading/1
  bank/1 -> Mux1/1
  pitch/1 -> Mux1/2
  heading/1 -> Mux1/3
  Mux1/1 -> Demux2/1, Demux1/1

== system Navion_6DoF_YANG/Aircraft_Dynamics/Equations of motion numerical integration /Moment Equations ==
  note: 1   c1
      | 2   c2
      | 3   c3
      | 4  c4
      | 5  c5
      | 6  c6
      | 7  c7
      | 8  c8
      | 9  c9
      | 10 Croll
      | 11  M
      | 12  N
      | 13  p
      | 14  q
      | 15  r
  note: p,q.r
  Inertia : Inport
  Moments : Inport  Port=2
  Demux1 : Demux  Outputs=3
      settings: DisplayOption=none
  Demux2 : Demux  Outputs=9
      settings: DisplayOption=none
  Demux3 : Demux  Outputs=3
      settings: DisplayOption=none
  Demux4 : Demux  Outputs=3
      settings: DisplayOption=none
  Inertia Coefs : Subsystem
  Mux : Mux  Inputs=15
  Mux1 : Mux  Inputs=3
  Mux2 : Mux  Inputs=3
  p integrate : Integrator  InitialCondition=initp
  pdot : Fcn  Expr=(u[1]*u[15]+u[2]*u[13])*u[14] + u[3]*u[10] + u[4]*u[12]
  q integrate : Integrator  InitialCondition=initq
  qdot : Fcn  Expr=u[5]*u[13]*u[15] - u[6]*(u[13]^2-u[15]^2) + u[7] * u[11]
  r integrate : Integrator  InitialCondition=initr
  rdot : Fcn  Expr=(u[8]*u[13]-u[2]*u[15]) * u[14] + u[4] * u[10] + u[9] * u[12]
  Ang Rates : Outport
  Ang Accel : Outport  Port=2
  wires:
  Inertia/1 -> Inertia Coefs/1(Inertia)
  Moments/1 -> Demux1/1
  Inertia Coefs/1(Iner Coef) -> Demux2/1
  Demux2/1 -> Mux/1
  Demux2/2 -> Mux/2
  Demux2/3 -> Mux/3
  Demux2/4 -> Mux/4
  Demux2/5 -> Mux/5
  Demux2/6 -> Mux/6
  Demux2/7 -> Mux/7
  Demux2/8 -> Mux/8
  Demux2/9 -> Mux/9
  Demux1/1 -> Mux/10
  Demux1/2 -> Mux/11
  Demux1/3 -> Mux/12
  Demux3/1 -> Mux/13
  Demux3/2 -> Mux/14
  Demux3/3 -> Mux/15
  Mux/1 -> pdot/1, qdot/1, rdot/1
  qdot/1 -> Mux1/2
  pdot/1 -> Mux1/1
  rdot/1 -> Mux1/3
  Mux1/1 -> Ang Accel/1, Demux4/1
  Demux4/1 -> p integrate/1
  Demux4/2 -> q integrate/1
  Demux4/3 -> r integrate/1
  Mux2/1 -> Ang Rates/1, Demux3/1
  p integrate/1 -> Mux2/1
  q integrate/1 -> Mux2/2
  r integrate/1 -> Mux2/3

== system Navion_6DoF_YANG/Aircraft_Dynamics/Linear Acc and Moments/Cross Prod Moment due to Aero ==
  Vec 1 : Inport
  Vec 2 : Inport  Port=2
  Demux : Demux  Outputs=3
      settings: DisplayOption=none
  Demux1 : Demux  Outputs=3
      settings: DisplayOption=none
  J axis : Fcn  Expr=u[4]*u[3] - u[6]*u[1]
  Mux : Mux  Inputs=6
  Mux1 : Mux  Inputs=3
  i axis : Fcn  Expr=u[6]*u[2] - u[5]*u[3]
  k axis : Fcn  Expr=u[5]*u[1] - u[4]*u[2]
  X Prod : Outport
  wires:
  Vec 2/1 -> Demux1/1
  Vec 1/1 -> Demux/1
  Demux/1 -> Mux/1
  Demux1/3 -> Mux/6
  Demux1/2 -> Mux/5
  Demux1/1 -> Mux/4
  Demux/3 -> Mux/3
  Demux/2 -> Mux/2
  Mux/1 -> i axis/1, J axis/1, k axis/1
  J axis/1 -> Mux1/2
  i axis/1 -> Mux1/1
  k axis/1 -> Mux1/3
  Mux1/1 -> X Prod/1

== system Navion_6DoF_YANG/Aircraft_Dynamics/Linear Acc and Moments/Left Cross Prod Moment due Leng ==
  Vec 1 : Inport
  Vec 2 : Inport  Port=2
  Check prob not zero : Constant  Value=0
  Demux : Demux  Outputs=3
      settings: DisplayOption=none
  J axis : Fcn  Expr=u[4]*u[3] - u[6]*u[1]
  Mux : Mux  Inputs=6
  Mux1 : Mux  Inputs=3
  i axis : Fcn  Expr=u[6]*u[2] - u[5]*u[3]
  k axis : Fcn  Expr=u[5]*u[1] - u[4]*u[2]
  X Prod : Outport
  wires:
  Vec 2/1 -> Mux/4
  Vec 1/1 -> Demux/1
  Demux/1 -> Mux/1
  Check prob not zero/1 -> Mux/5, Mux/6
  Demux/3 -> Mux/3
  Demux/2 -> Mux/2
  Mux/1 -> J axis/1, k axis/1, i axis/1
  J axis/1 -> Mux1/2
  i axis/1 -> Mux1/1
  k axis/1 -> Mux1/3
  Mux1/1 -> X Prod/1

== system Navion_6DoF_YANG/Aircraft_Dynamics/Linear Acc and Moments/Right Cross Prod Moment due Leng1 ==
  Vec 1 : Inport
  Vec 2 : Inport  Port=2
  Check prob not zero : Constant  Value=0
  Demux : Demux  Outputs=3
      settings: DisplayOption=none
  J axis : Fcn  Expr=u[4]*u[3] - u[6]*u[1]
  Mux : Mux  Inputs=6
  Mux1 : Mux  Inputs=3
  i axis : Fcn  Expr=u[6]*u[2] - u[5]*u[3]
  k axis : Fcn  Expr=u[5]*u[1] - u[4]*u[2]
  X Prod : Outport
  wires:
  Vec 2/1 -> Mux/4
  Vec 1/1 -> Demux/1
  Demux/1 -> Mux/1
  Check prob not zero/1 -> Mux/5, Mux/6
  Demux/3 -> Mux/3
  Demux/2 -> Mux/2
  Mux/1 -> i axis/1, J axis/1, k axis/1
  J axis/1 -> Mux1/2
  i axis/1 -> Mux1/1
  k axis/1 -> Mux1/3
  Mux1/1 -> X Prod/1

== system Navion_6DoF_YANG/Aircraft_Dynamics/Aerodynamics/Aero Forces and Moments/Aerodynamic Forces ==
  CD : Inport
  CY : Inport  Port=2
  CL : Inport  Port=3
  Wind Para : Inport  Port=4
  dyn(q) : Inport  Port=5
  Body to Wind : Subsystem
  Demux : Demux  Outputs=3
      settings: DisplayOption=none
  Gain : Gain  Gain=-1  SaturateOnIntegerOverflow=on  OutDataTypeStr=Inherit: Same as input  ParamDataTypeStr=Inherit: Same as input
  Gain1 : Gain  Gain=-1  SaturateOnIntegerOverflow=on  OutDataTypeStr=Inherit: Same as input  ParamDataTypeStr=Inherit: Same as input
  Gain2 : Gain  Gain=sw  SaturateOnIntegerOverflow=on  OutDataTypeStr=Inherit: Same as input  ParamDataTypeStr=Inherit: Same as input
  Math Function : Math  Operator=transpose  SignedPower=on  SaturateOnIntegerOverflow=on
  Mux : Mux  Inputs=3
  Product : Product  SaturateOnIntegerOverflow=on  OutDataTypeStr=Inherit: Same as first input
  Product1 : Product  Multiplication=Matrix(*)  SaturateOnIntegerOverflow=on  OutDataTypeStr=Inherit: Same as first input
  Terminator : Terminator
  FaeroBody : Outport
  wires:
  Gain/1 -> Mux/1
  Gain1/1 -> Mux/3
  Mux/1 -> Product/1
  Gain2/1 -> Product/2
  CD/1 -> Gain/1
  CY/1 -> Mux/2
  CL/1 -> Gain1/1
  dyn(q)/1 -> Gain2/1
  Wind Para/1 -> Demux/1
  Demux/1 -> Terminator/1
  Body to Wind/1(Smatrix) -> Math Function/1
  Math Function/1 -> Product1/1
  Product/1 -> Product1/2
  Product1/1 -> FaeroBody/1
  Demux/2 -> Body to Wind/1(Alpha)
  Demux/3 -> Body to Wind/2(Beta)

== system Navion_6DoF_YANG/Aircraft_Dynamics/Aerodynamics/Aero Forces and Moments/Aerodynamic Moments ==
  dyn(q) : Inport
  Croll : Inport  Port=2
  CM : Inport  Port=3
  CN : Inport  Port=4
  Mux : Mux  Inputs=2
  Mux1 : Mux  Inputs=2
  Mux2 : Mux  Inputs=2
  Mux3 : Mux  Inputs=3
  Pitch : Fcn  Expr=u[1] * sw * cbar * u[2]
  Roll : Fcn  Expr=u[1] * sw * b * u[2]
  Yaw : Fcn  Expr=u[1] * sw * b * u[2]
  Maero : Outport
  wires:
  Mux/1 -> Roll/1
  Mux1/1 -> Pitch/1
  Mux2/1 -> Yaw/1
  Pitch/1 -> Mux3/2
  Roll/1 -> Mux3/1
  Yaw/1 -> Mux3/3
  dyn(q)/1 -> Mux/1, Mux1/1, Mux2/1
  Croll/1 -> Mux/2
  CM/1 -> Mux1/2
  CN/1 -> Mux2/2
  Mux3/1 -> Maero/1

== system Navion_6DoF_YANG/Aircraft_Dynamics/Aerodynamics/CD/Get Alpha ==
  windPar : Inport
  "   " : Terminator
  "   1" : Terminator
  Demux : Demux  Outputs=3
      settings: DisplayOption=none
  Alpha : Outport
  wires:
  Demux/1 -> "   1"/1
  Demux/3 -> "   "/1
  windPar/1 -> Demux/1
  Demux/2 -> Alpha/1

== system Navion_6DoF_YANG/Aircraft_Dynamics/Engines/Lycoming IO-Left/Prop Efficiency  with Cp input ==
  TAS : Inport
  RPS : Inport  Port=2
  Prop D : Inport  Port=3
  CP table : Constant  Value=CP_norm
  Eff vs J : Lookup2D  RowIndex=PropEff_norm(:,1)  ColumnIndex=pitch_Angles  Table=PropEff_norm(:,2:7)  LookUpMeth=Interpolation-Use End Values
  Embedded MATLAB Function Retrieving Pich Angle : MATLAB Function  TreatAsAtomicUnit=on
  J : Fcn  Expr=u(1)/(u(2)*u(3))
  J2 : Display
  Mux3 : Mux  Inputs=3
  Mux5 : Mux  Inputs=2
  efficiency : Display
  efficiency comp : Scope
  pitch : Display
  n : Outport
  wires:
  Prop D/1 -> Mux3/3
  RPS/1 -> Mux3/2
  TAS/1 -> Mux3/1
  J/1 -> J2/1, Eff vs J/1, Embedded MATLAB Function Retrieving Pich Angle/2(j)
  CP table/1 -> Embedded MATLAB Function Retrieving Pich Angle/3(CP_norm)
  Embedded MATLAB Function Retrieving Pich Angle/1(Pitch) -> pitch/1, Eff vs J/2
  Eff vs J/1 -> n/1, Mux5/2, efficiency/1
  [Cp_left] -> Embedded MATLAB Function Retrieving Pich Angle/1(CP)
  Mux5/1 -> efficiency comp/1
  [n_FTD] -> Mux5/1
  Mux3/1 -> J/1

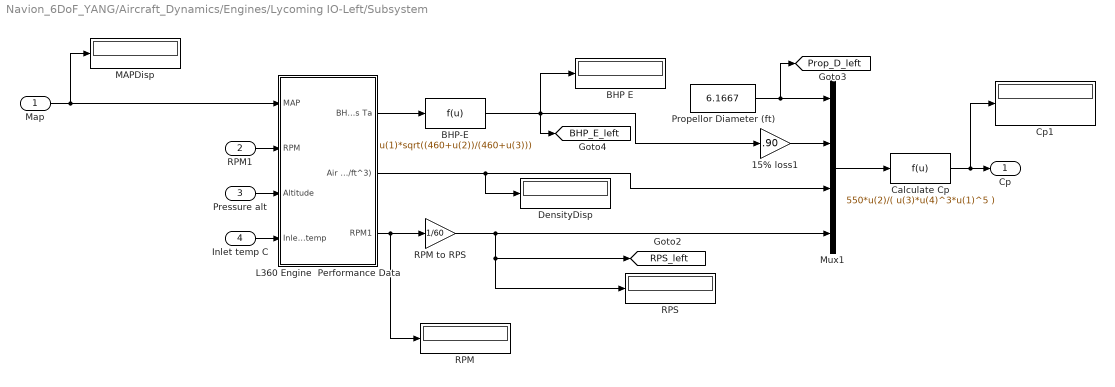
== system Navion_6DoF_YANG/Aircraft_Dynamics/Engines/Lycoming IO-Left/Subsystem ==
  Map : Inport
  RPM1 : Inport  Port=2
  Pressure alt : Inport  Port=3
  Inlet temp C : Inport  Port=4
  15% loss1 : Gain  Gain=.90
  BHP E : Display
  BHP-E : Fcn  Expr=u(1)*sqrt((460+u(2))/(460+u(3)))
  Calculate Cp : Fcn  Expr=550*u(2)/( u(3)*u(4)^3*u(1)^5 )
  Cp1 : Display
  DensityDisp : Display
  L360 Engine  Performance Data : Subsystem
  MAPDisp : Display
  Mux1 : Mux
  Propellor Diameter (ft) : Constant  Value=6.1667
  RPM : Display
  "RPM to RPS " : Gain  Gain=1/60
  RPS : Display
  Cp : Outport
  tag scope: BHP_E_left=global, Prop_D_left=global, RPS_left=global
  wires:
  Inlet temp C/1 -> L360 Engine  Performance Data/4(Inlet air temp)
  Pressure alt/1 -> L360 Engine  Performance Data/3(Altitude)
  RPM1/1 -> L360 Engine  Performance Data/2(RPM)
  15% loss1/1 -> Mux1/2
  BHP-E/1 -> 15% loss1/1, [BHP_E_left], BHP E/1
  Calculate Cp/1 -> Cp/1, Cp1/1
  "RPM to RPS "/1 -> [RPS_left], RPS/1, Mux1/4
  L360 Engine  Performance Data/3(RPM1) -> RPM/1, "RPM to RPS "/1
  L360 Engine  Performance Data/2(Air Density (slugs/ft^3)) -> DensityDisp/1, Mux1/3
  Mux1/1 -> Calculate Cp/1
  Propellor Diameter (ft)/1 -> [Prop_D_left], Mux1/1
  L360 Engine  Performance Data/1(BHP-D Ts Ta) -> BHP-E/1
  Map/1 -> L360 Engine  Performance Data/1(MAP), MAPDisp/1

== system Navion_6DoF_YANG/Aircraft_Dynamics/Engines/Lycoming IO-Left/Thrust ==
  TAS : Inport
  BHP E : Inport  Port=2
  n : Inport  Port=3
  # eng : Gain
  15% loss : Gain  Gain=.90
  15% loss2 : Gain
  15% loss4 : Gain
  Convert to Thrust : Fcn  Expr=(550*u(3)*u(2)/u(1))
  Mux2 : Mux  Inputs=3
  Thrust : Display
  "thrust " : Outport
  wires:
  n/1 -> Mux2/3
  BHP E/1 -> 15% loss/1
  TAS/1 -> 15% loss2/1
  # eng/1 -> "thrust "/1
  15% loss4/1 -> # eng/1, Thrust/1
  15% loss2/1 -> Mux2/1
  15% loss/1 -> Mux2/2
  Convert to Thrust/1 -> 15% loss4/1
  Mux2/1 -> Convert to Thrust/1

== system Navion_6DoF_YANG/Aircraft_Dynamics/Engines/Lycoming IO-Right/Prop Efficiency  with Cp input ==
  TAS : Inport
  RPS : Inport  Port=2
  Prop D : Inport  Port=3
  CP table : Constant  Value=CP_norm
  Eff vs J : Lookup2D  RowIndex=PropEff_norm(:,1)  ColumnIndex=pitch_Angles  Table=PropEff_norm(:,2:7)  LookUpMeth=Interpolation-Use End Values
  Embedded MATLAB Function Retrieving Pich Angle : MATLAB Function  TreatAsAtomicUnit=on
  J : Fcn  Expr=u(1)/(u(2)*u(3))
  J2 : Display
  Mux3 : Mux  Inputs=3
  Mux5 : Mux  Inputs=2
  efficiency : Display
  efficiency comp : Scope
  pitch : Display
  n : Outport
  wires:
  Prop D/1 -> Mux3/3
  RPS/1 -> Mux3/2
  TAS/1 -> Mux3/1
  J/1 -> J2/1, Eff vs J/1, Embedded MATLAB Function Retrieving Pich Angle/2(j)
  CP table/1 -> Embedded MATLAB Function Retrieving Pich Angle/3(CP_norm)
  Embedded MATLAB Function Retrieving Pich Angle/1(Pitch) -> pitch/1, Eff vs J/2
  Eff vs J/1 -> n/1, Mux5/2, efficiency/1
  [Cp_right] -> Embedded MATLAB Function Retrieving Pich Angle/1(CP)
  Mux5/1 -> efficiency comp/1
  [n_FTD] -> Mux5/1
  Mux3/1 -> J/1

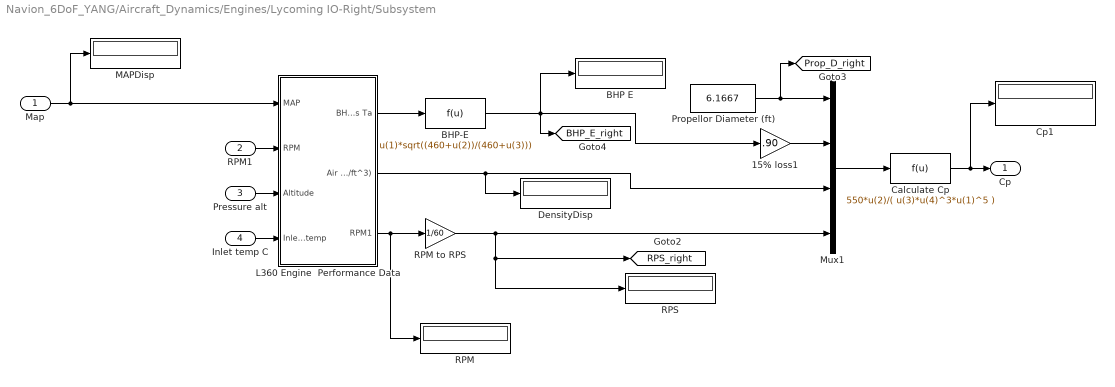
== system Navion_6DoF_YANG/Aircraft_Dynamics/Engines/Lycoming IO-Right/Subsystem ==
  Map : Inport
  RPM1 : Inport  Port=2
  Pressure alt : Inport  Port=3
  Inlet temp C : Inport  Port=4
  15% loss1 : Gain  Gain=.90
  BHP E : Display
  BHP-E : Fcn  Expr=u(1)*sqrt((460+u(2))/(460+u(3)))
  Calculate Cp : Fcn  Expr=550*u(2)/( u(3)*u(4)^3*u(1)^5 )
  Cp1 : Display
  DensityDisp : Display
  L360 Engine  Performance Data : Subsystem
  MAPDisp : Display
  Mux1 : Mux
  Propellor Diameter (ft) : Constant  Value=6.1667
  RPM : Display
  "RPM to RPS " : Gain  Gain=1/60
  RPS : Display
  Cp : Outport
  tag scope: BHP_E_right=global, Prop_D_right=global, RPS_right=global
  wires:
  Inlet temp C/1 -> L360 Engine  Performance Data/4(Inlet air temp)
  Pressure alt/1 -> L360 Engine  Performance Data/3(Altitude)
  RPM1/1 -> L360 Engine  Performance Data/2(RPM)
  15% loss1/1 -> Mux1/2
  BHP-E/1 -> 15% loss1/1, [BHP_E_right], BHP E/1
  Calculate Cp/1 -> Cp/1, Cp1/1
  "RPM to RPS "/1 -> [RPS_right], RPS/1, Mux1/4
  L360 Engine  Performance Data/3(RPM1) -> RPM/1, "RPM to RPS "/1
  L360 Engine  Performance Data/2(Air Density (slugs/ft^3)) -> DensityDisp/1, Mux1/3
  Mux1/1 -> Calculate Cp/1
  Propellor Diameter (ft)/1 -> [Prop_D_right], Mux1/1
  L360 Engine  Performance Data/1(BHP-D Ts Ta) -> BHP-E/1
  Map/1 -> L360 Engine  Performance Data/1(MAP), MAPDisp/1

== system Navion_6DoF_YANG/Aircraft_Dynamics/Engines/Lycoming IO-Right/Thrust ==
  TAS : Inport
  BHP E : Inport  Port=2
  n : Inport  Port=3
  # eng : Gain
  15% loss : Gain  Gain=.90
  15% loss2 : Gain
  15% loss4 : Gain
  Convert to Thrust : Fcn  Expr=(550*u(3)*u(2)/u(1))
  Mux2 : Mux  Inputs=3
  Thrust : Display
  "thrust " : Outport
  wires:
  n/1 -> Mux2/3
  BHP E/1 -> 15% loss/1
  TAS/1 -> 15% loss2/1
  # eng/1 -> "thrust "/1
  15% loss4/1 -> # eng/1, Thrust/1
  15% loss2/1 -> Mux2/1
  15% loss/1 -> Mux2/2
  Convert to Thrust/1 -> 15% loss4/1
  Mux2/1 -> Convert to Thrust/1

== system Navion_6DoF_YANG/Aircraft_Dynamics/Equations of motion numerical integration /Kinematic Equiations/2pi Bound ==
  In : Inport
  2pi : Constant  Value=2*pi
  Math Function : Math  Operator=mod  SignedPower=on  SaturateOnIntegerOverflow=on
  Out : Outport
  wires:
  Math Function/1 -> Out/1
  2pi/1 -> Math Function/2
  In/1 -> Math Function/1

== system Navion_6DoF_YANG/Aircraft_Dynamics/Equations of motion numerical integration /Kinematic Equiations/pi Bound ==
  In : Inport
  2pi : Constant  Value=2*pi
  Math Function : Math  Operator=mod  SignedPower=on  SaturateOnIntegerOverflow=on
  Sum1 : Sum  Inputs=|+-  InputSameDT=on  SaturateOnIntegerOverflow=on  OutDataTypeStr=Inherit: Same as first input
  Sum2 : Sum  Inputs=|++  InputSameDT=on  SaturateOnIntegerOverflow=on  OutDataTypeStr=Inherit: Same as first input
  pi : Constant  Value=pi
  Out : Outport
  wires:
  Sum1/1 -> Out/1
  pi/1 -> Sum1/2, Sum2/2
  Sum2/1 -> Math Function/1
  In/1 -> Sum2/1
  2pi/1 -> Math Function/2
  Math Function/1 -> Sum1/1

== system Navion_6DoF_YANG/Aircraft_Dynamics/Equations of motion numerical integration /Kinematic Equiations/pi Bound1 ==
  In : Inport
  2pi : Constant  Value=2*pi
  Math Function : Math  Operator=mod  SignedPower=on  SaturateOnIntegerOverflow=on
  Sum1 : Sum  Inputs=|+-  InputSameDT=on  SaturateOnIntegerOverflow=on  OutDataTypeStr=Inherit: Same as first input
  Sum2 : Sum  Inputs=|++  InputSameDT=on  SaturateOnIntegerOverflow=on  OutDataTypeStr=Inherit: Same as first input
  pi : Constant  Value=pi
  Out : Outport
  wires:
  Sum1/1 -> Out/1
  pi/1 -> Sum1/2, Sum2/2
  Sum2/1 -> Math Function/1
  In/1 -> Sum2/1
  2pi/1 -> Math Function/2
  Math Function/1 -> Sum1/1

== system Navion_6DoF_YANG/Aircraft_Dynamics/Equations of motion numerical integration /Moment Equations/Inertia Coefs ==
  note: Jx,Jy,Jz,Jxz
  note: Inertia Coefficeents
      | Page 80 Stevens and Lewis
  Inertia : Inport
  Mux : Mux  Inputs=9
  c1 : Fcn  Expr=((u[2]-u[3])*u[3] - u[4]^2)/(u[1]*u[3]-u[4]^2)
  c2 : Fcn  Expr=((u[1]-u[2]+u[3])*u[4])/(u[1]*u[3]-u[4]^2)
  c3 : Fcn  Expr=u[3]/(u[1]*u[3]-u[4]^2)
  c4 : Fcn  Expr=u[4]/(u[1]*u[3]-u[4]^2)
  c5 : Fcn  Expr=(u[3]-u[1])/u[2]
  c6 : Fcn  Expr=u[4]/u[2]
  c7 : Fcn  Expr=1/u[2]
  c8 : Fcn  Expr=(u[1]*(u[1]-u[2])+u[4]^2)/(u[1]*u[3]-u[4]^2)
  c9 : Fcn  Expr=u[1]/(u[1]*u[3]-u[4]^2)
  Iner Coef : Outport
  wires:
  Inertia/1 -> c1/1, c2/1, c3/1, c4/1, c5/1, c6/1, c7/1, c9/1, c8/1
  c1/1 -> Mux/1
  c2/1 -> Mux/2
  c3/1 -> Mux/3
  c4/1 -> Mux/4
  c5/1 -> Mux/5
  c6/1 -> Mux/6
  c7/1 -> Mux/7
  c8/1 -> Mux/8
  c9/1 -> Mux/9
  Mux/1 -> Iner Coef/1
